simulink model "Adjust"  (R2016b)
settings: Solver=VariableStepAuto  StartTime=0.0  StopTime=5.0  RelTol=1e-3
undefined symbols (not defined in the file): CR, LF, serial
libraries: instrumentlib x3
settings Model: Creator=oscar  LastModifiedBy=oscar

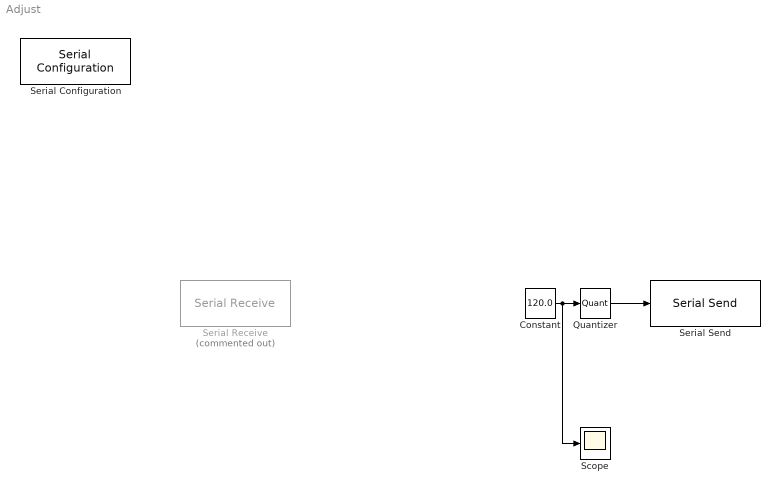
== system Adjust ==
  Constant : Constant  Value=120.0  OutDataTypeStr=double  SampleTime=1
  Quantizer : Quantizer
  Scope : Scope
  Serial Configuration : instrumentlib/Serial Configuration  Priority=-200000  ComPortMenu=<Please select a port...>  ComPort=/dev/ttyUSB0  ObjConstructor=serial('/dev/ttyUSB0');  BaudRate=115200  DataBits=8  Parity=none  StopBits=1  FlowControl=none  Timeout=10  ByteOrder=LittleEndian
  Serial Receive : instrumentlib/Serial Receive  Commented=on  ComPortMenu=<Please select a port...>  ComPort=/dev/ttyUSB0  ObjConstructor=serial('/dev/ttyUSB0');  Terminator=CR/LF ('\r\n')  DataSize=1  DataType=single  EnableBlockingMode=on  ActionDataUnavailable=Output last received value  CustomValue=0  SampleTime=0.1
  Serial Send : instrumentlib/Serial Send  ComPortMenu=/dev/ttyUSB0  ComPort=/dev/ttyUSB0  ObjConstructor=serial('/dev/ttyUSB0');  Terminator=LF ('\n')  EnableBlockingMode=on
  wires:
  Quantizer/1 -> Serial Send/1
  Constant/1 -> Scope/1, Quantizer/1
